simulink model "ee_motor_pmsm_drive_noContr"  (R2021b)
settings: Solver=ode23t  StartTime=0.0  StopTime=tsim  FixedStep=Ts  MaxStep=1e-6  RelTol=1e-4  AbsTol=1e-3  EnableMultiTasking=on
values from neighbouring files (symbols this model uses):
  angleVec = [0 1 2 3 4 5 6 7 8 9 10 11 ... (31 elements, 1x31)]    [currentsDQ_LUT.mat]    (also in di_pmsm_model_generator.m = [0:1:90]; di_pmsm_model_motor.m = [0:1:90])
  fsw = 2e3    (= 2000)    [ee_motor_pmsm_drive_noContr_params.m]    (also in ee_motor_pmsm_drive_test_params.m = 20000)
  Imax = 1000    [ee_motor_pmsm_drive_noContr_params.m]    (also in ee_motor_pmsm_drive_test_params.m = 320)
  J = 0.02    [di_pmsm_model_MPC.m]    (also in di_pmsm_model_generator_invLUT_V2.m; ee_motor_pmsm_drive_noContr_params.m)
  Ld = 0.0013    [di_pmsm_model_MPC.m]    (also in di_pmsm_model_generator_idealMod.m = (mean(dflux(p60_idx,:))-mean(dflux(m90_idx,:)))/(60-(-90)); ee_4d_table.m = 0.0002; ee_motor_pmsm_drive_noContr_params.m; ee_motor_pmsm_drive_test_params.m)
  Lq = 0.0039    [di_pmsm_model_MPC.m]    (also in di_pmsm_model_generator_idealMod.m = (mean(fq(p30_idx,:))-mean(fq(m30_idx,:)))/(30-(-30)); ee_4d_table.m = 0.0005; ee_motor_pmsm_drive_noContr_params.m; ee_motor_pmsm_drive_test_params.m)
  N = 4    [ee_4d_table.m]    (also in flux_derivatives_test.m = 6)
  PM = 0.1571    [di_pmsm_model_MPC.m]    (also in di_pmsm_model_generator_idealMod.m = fd_0; ee_4d_table.m = 0.1; ee_motor_pmsm_drive_noContr_params.m; ee_motor_pmsm_drive_test_params.m)
  rpm0 = 7200    [ee_motor_pmsm_drive_noContr_params.m]    (also in ee_motor_pmsm_drive_test_params.m = rpm_nom)
  Rs = 0.013    [ee_4d_table.m]    (also in ee_motor_pmsm_drive_noContr_params.m = 0.07; ee_motor_pmsm_drive_test_params.m = 0.07; flux_derivatives_test.m)
  Tmax = 460    [di_pmsm_model_MPC.m]    (also in ee_motor_pmsm_drive_noContr_params.m = 1.5*N*PM*Imax; ee_motor_pmsm_drive_test_params.m = 1.5*N*PM*Imax)
  torque = [461.04655919 409.33694322 395.67421775 372.972407 342.22869649 310.06846718 277.66285866 246.48195035 220.59637081 202.25585677 184.09571331 161.22594217 ... (40131 elements, 21x21x91)]    [torqueDQ_LUT_new.mat]
  torque0 = 0    [ee_motor_pmsm_drive_noContr_params.m]    (also in ee_motor_pmsm_drive_test_params.m)
  Ts = 1e-6    (= 1e-06)    [PruebaRN.m]    (also in di_pmsm_model_generator.m; di_pmsm_model_generator_idealMod.m; di_pmsm_model_generator_invLUT.m; di_pmsm_model_generator_invLUT_V2.m)
  Tsc = 1/fc    (= 5e-05)    [ee_motor_pmsm_drive_noContr_params.m]    (also in ee_motor_pmsm_drive_test_params.m = 5e-06)
  Vdc = 50    [ee_motor_pmsm_drive_noContr_params.m]
undefined symbols (not defined in the file or in its folder): data, idVec, iqVec, kif, kin, kit, kpf, kpn, kpt, vpor
libraries: simulink_need_slupdate x3, eeTransforms x3, slpidlib x3, eePwmGeneratorTwoLevel x1, simulink x1
Description:
  | HEV PMSM Drive Test Harness
settings Model: Creator=The MathWorks, Inc.  LastModifiedBy=crist
settings SolverCC: AutoScaleAbsTol=off  MaxConsecutiveMinStep=2  AlgebraicLoopSolver=TrustRegion
settings DataIOCC: LimitDataPoints=on  MaxDataPoints=35000  SaveFormat=StructureWithTime  SaveOutput=off  DSMLogging=off  ReturnWorkspaceOutputs=off  SignalLoggingName=logsout_ee_motor_pmsm_drive
settings OptimizationCC: LifeSpan=inf
settings DebuggingCC: UnderspecifiedInitializationDetection=Classic  MergeDetectMultiDrivingBlocksExec=none  AllowSymbolicDim=off  PregeneratedLibrarySubsystemCodeDiagnostic=none  SFUnexpectedBacktrackingDiag=warning  SFNoUnconditionalDefaultTransitionDiag=warning  SFExecutionAtInitializationDiag=none  SFMachineParentedDataDiag=warning  ArithmeticOperatorsInVariantConditions=warning
settings HardwareCC: ProdBitPerPointer=32  ProdBitPerSizeT=32  ProdBitPerPtrDiffT=32  ProdLargestAtomicFloat=None  ProdIntDivRoundTo=Undefined  ProdEndianess=Unspecified  ProdWordSize=32  ProdHWDeviceType=32-bit Generic
settings ModelReferenceCC: PropagateSignalLabelsOutOfModel=off
settings SFSimCC: SimUseLocalCustomCode=off
settings RTWCC: RTWUseLocalCustomCode=off
settings CodeAppCC: StateflowObjectComments=on
settings GRTTargetCC: TargetLangStandard=C89/C90 (ANSI)
settings ConfigComp: CovMetricSettings=dw  CovSaveCumulativeToWorkspaceVar=on  CovSaveSingleToWorkspaceVar=on  CovExternalEMLEnable=off  CovSFcnEnable=off
settings SimscapeCC: SimscapeLogType=all  SimscapeLogSimulationStatistics=on  SimscapeLogName=simlog_ee_motor_pmsm_drive  SimscapeLogDecimation=10  SimscapeLogLimitData=off  SimscapeLogDataHistory=1000000

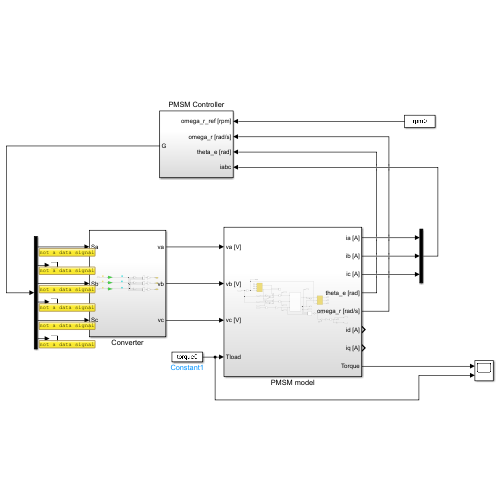
[thumbnail: Simulink's stored preview of the top-level diagram]
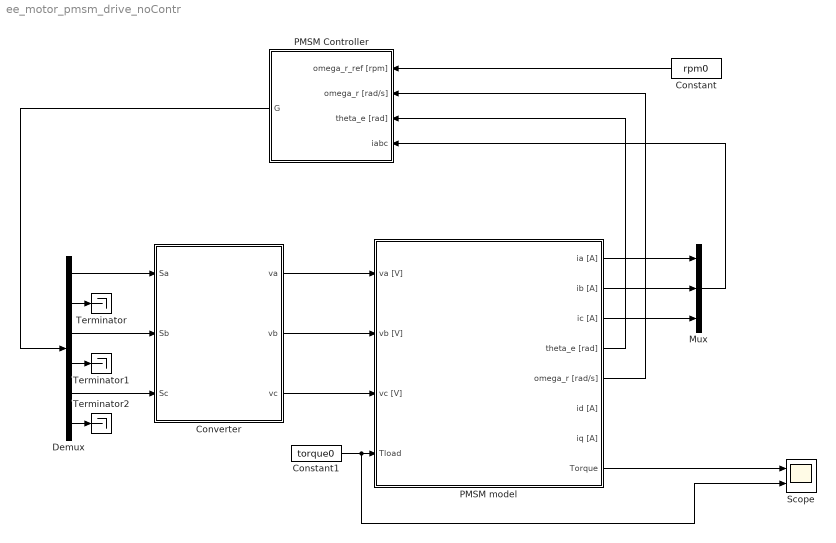
== system ee_motor_pmsm_drive_noContr ==
  Constant : Constant  Value=rpm0
  Constant1 : Constant  Value=torque0
  Converter : Subsystem
  Demux : Demux  Outputs=6
  Mux : Mux  Inputs=3
  PMSM Controller : Subsystem
  PMSM model : Subsystem
  Scope : Scope  NumInputPorts=2
  Terminator : Terminator
  Terminator1 : Terminator
  Terminator2 : Terminator
  wires:
  PMSM model/2(ib [A]) -> Mux/2
  PMSM model/1(ia [A]) -> Mux/1
  PMSM model/3(ic [A]) -> Mux/3
  Mux/1 -> PMSM Controller/4(iabc)
  Constant1/1 -> Scope/2, PMSM model/4(Tload)
  Constant/1 -> PMSM Controller/1(omega_r_ref [rpm])
  PMSM model/5(omega_r [rad/s]) -> PMSM Controller/2(omega_r [rad/s])
  PMSM model/4(theta_e [rad]) -> PMSM Controller/3(theta_e [rad])
  Converter/1(va) -> PMSM model/1(va [V])
  Converter/3(vc) -> PMSM model/3(vc [V])
  Converter/2(vb) -> PMSM model/2(vb [V])
  Demux/1 -> Converter/1(Sa)
  PMSM Controller/1(G) -> Demux/1
  Demux/3 -> Converter/2(Sb)
  Demux/5 -> Converter/3(Sc)
  Demux/2 -> Terminator/1
  Demux/4 -> Terminator1/1
  Demux/6 -> Terminator2/1
  PMSM model/8(Torque) -> Scope/1

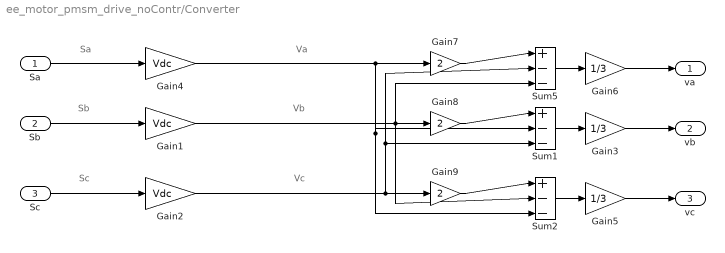
== system ee_motor_pmsm_drive_noContr/Converter ==
  note: Vb
  note: Sa
  note: Sc
  note: Va
  note: Vc
  note: Sb
  Sa : Inport
  Sb : Inport  Port=2
  Sc : Inport  Port=3
  Gain1 : Gain  Gain=Vdc
  Gain2 : Gain  Gain=Vdc
  Gain3 : Gain  Gain=1/3
  Gain4 : Gain  Gain=Vdc
  Gain5 : Gain  Gain=1/3
  Gain6 : Gain  Gain=1/3
  Gain7 : Gain  Gain=2
  Gain8 : Gain  Gain=2
  Gain9 : Gain  Gain=2
  Sum1 : Sum  Inputs=|+--
  Sum2 : Sum  Inputs=|+--
  Sum5 : Sum  Inputs=|+--
  va : Outport
  vb : Outport  Port=2
  vc : Outport  Port=3
  wires:
  Gain2/1 -> Gain9/1, Sum5/2, Sum1/3
  Gain9/1 -> Sum2/1
  Sum2/1 -> Gain5/1
  Gain4/1 -> Gain7/1, Sum1/2, Sum2/3
  Sum5/1 -> Gain6/1
  Gain7/1 -> Sum5/1
  Gain8/1 -> Sum1/1
  Sb/1 -> Gain1/1
  Gain6/1 -> va/1
  Gain5/1 -> vc/1
  Sum1/1 -> Gain3/1
  Gain3/1 -> vb/1
  Sc/1 -> Gain2/1
  Sa/1 -> Gain4/1
  Gain1/1 -> Gain8/1, Sum5/3, Sum2/2

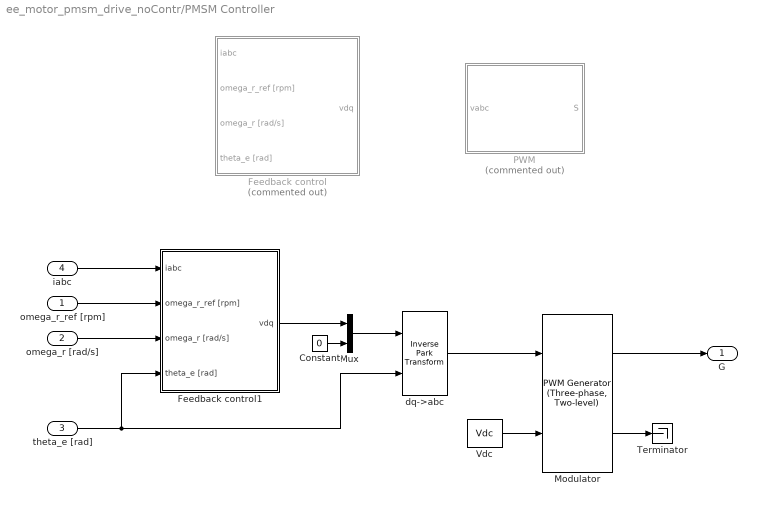
== system ee_motor_pmsm_drive_noContr/PMSM Controller ==
  omega_r_ref [rpm] : Inport
  omega_r [rad/s] : Inport  Port=2
  theta_e [rad] : Inport  Port=3
  iabc : Inport  Port=4
  Constant : Constant  Value=0  SampleTime=-1
  Feedback control : Subsystem  Commented=on
  Feedback control1 : Subsystem
  Modulator : eePwmGeneratorTwoLevel/PWM Generator (Three-phase, Two-level)  PWMMode=Continuous PWM (CPWM)  CPWMMode=SPWM: sinusoidal PWM  DPWMMode=60 DPWM: 60 degree discontinuous PWM  fsw=fsw  Ts=Ts
      settings: SourceProductBaseCode=PS
  Mux : Mux  Inputs=2
  PWM : Subsystem  Commented=on
  Terminator : Terminator
  Vdc : Constant  Value=Vdc  SampleTime=Tsc
  dq->abc : eeTransforms/Inverse Park Transform  AxisAlignment=Q-axis  PowerInvariant=off
  G : Outport  VectorParamsAs1DForOutWhenUnconnected=off
  wires:
  Vdc/1 -> Modulator/2
  Modulator/2 -> Terminator/1
  Modulator/1 -> G/1
  Constant/1 -> Mux/2
  Mux/1 -> dq->abc/1
  dq->abc/1 -> Modulator/1
  theta_e [rad]/1 -> Feedback control1/4(theta_e [rad]), dq->abc/2
  Feedback control1/1(vdq) -> Mux/1
  iabc/1 -> Feedback control1/1(iabc)
  omega_r_ref [rpm]/1 -> Feedback control1/2(omega_r_ref [rpm])
  omega_r [rad/s]/1 -> Feedback control1/3(omega_r [rad/s])

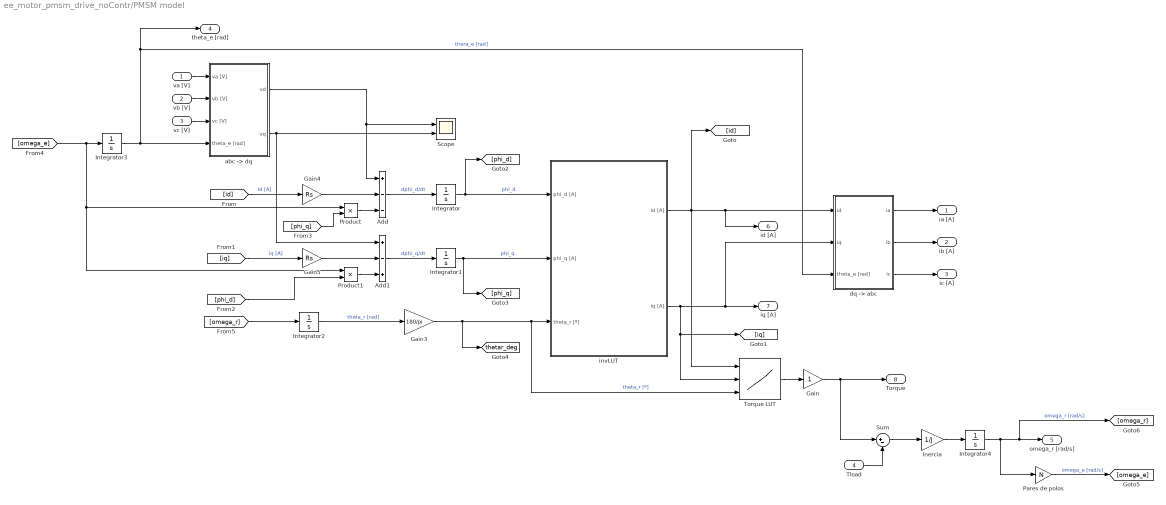
== system ee_motor_pmsm_drive_noContr/PMSM model ==
  va [V] : Inport
  vb [V] : Inport  Port=2
  vc [V] : Inport  Port=3
  Tload : Inport  Port=4
  Add : Sum  Inputs=+--
  Add1 : Sum  Inputs=+-+
  Gain : Gain
  Gain3 : Gain  Gain=180/pi
  Gain4 : Gain  Gain=Rs
  Gain5 : Gain  Gain=Rs
  Inercia : Gain  Gain=1/J
  Integrator : Integrator  InitialCondition=-0.2
  Integrator1 : Integrator
  Integrator2 : Integrator  WrapState=on  WrappedStateUpperValue=2*pi/3/N  WrappedStateLowerValue=0
  Integrator3 : Integrator
  Integrator4 : Integrator  InitialCondition=750
  Pares de polos : Gain  Gain=N
  Product : Product
  Product1 : Product
  Scope : Scope  NumInputPorts=2
  Sum : Sum  Inputs=|+-
  Torque LUT : Lookup_n-D  NumberOfTableDimensions=3  LookupTableObject=iD  BreakpointsForDimension1=idVec  BreakpointsForDimension2=iqVec  BreakpointsForDimension3=angleVec  Table=torque  InternalRulePriority=Speed  RndMeth=Simplest  InputSameDT=on
      settings: InputPortMap=u0,u1,u2
  "abc -> dq" : Subsystem
  "dq -> abc" : Subsystem
  "invLUT " : Subsystem
  ia [A] : Outport
  ib [A] : Outport  Port=2
  ic [A] : Outport  Port=3
  theta_e [rad] : Outport  Port=4
  omega_r [rad/s] : Outport  Port=5
  id [A] : Outport  Port=6
  iq [A] : Outport  Port=7
  Torque : Outport  Port=8
  tag scope: thetar_deg=global
  wires:
  Product/1 -> Add/3
  Integrator1/1 -> [phi_q], "invLUT "/2(phi_q [A])  "phi_q"
  [phi_q] -> Product/2
  [omega_e] -> Product/1, Product1/1, Integrator3/1
  Add/1 -> Integrator/1  "dphi_d/dt"
  [id] -> Gain4/1  "id [A]"
  Product1/1 -> Add1/3
  "invLUT "/1(id [A]) -> "dq -> abc"/1(id), id [A]/1, Torque LUT/1, [id]
  Integrator/1 -> "invLUT "/1(phi_d [A]), [phi_d]  "phi_d"
  "invLUT "/2(iq [A]) -> Torque LUT/2, [iq], "dq -> abc"/2(iq), iq [A]/1
  Add1/1 -> Integrator1/1  "dphi_q/dt"
  Gain5/1 -> Add1/2
  Gain4/1 -> Add/2
  "abc -> dq"/2(vq) -> Add1/1, Scope/2
  [iq] -> Gain5/1  "iq [A]"
  [phi_d] -> Product1/2
  "abc -> dq"/1(vd) -> Scope/1, Add/1
  va [V]/1 -> "abc -> dq"/1(va [V])
  vb [V]/1 -> "abc -> dq"/2(vb [V])
  vc [V]/1 -> "abc -> dq"/3(vc [V])
  Gain3/1 -> [thetar_deg], Torque LUT/3, "invLUT "/3(theta_r [º])  "theta_r [º]"
  [omega_r] -> Integrator2/1
  "dq -> abc"/1(ia) -> ia [A]/1
  "dq -> abc"/2(ib) -> ib [A]/1
  "dq -> abc"/3(ic) -> ic [A]/1
  Integrator2/1 -> Gain3/1  "theta_r [rad]"
  Integrator3/1 -> theta_e [rad]/1, "dq -> abc"/3(theta_e [rad]), "abc -> dq"/4(theta_e [rad])  "thera_e [rad]"
  Gain/1 -> Torque/1, Sum/1
  Pares de polos/1 -> [omega_e]  "omega_e [rad/s]"
  Sum/1 -> Inercia/1
  Inercia/1 -> Integrator4/1
  Integrator4/1 -> omega_r [rad/s]/1, [omega_r], Pares de polos/1  "omega_r [rad/s]"
  Tload/1 -> Sum/2
  Torque LUT/1 -> Gain/1

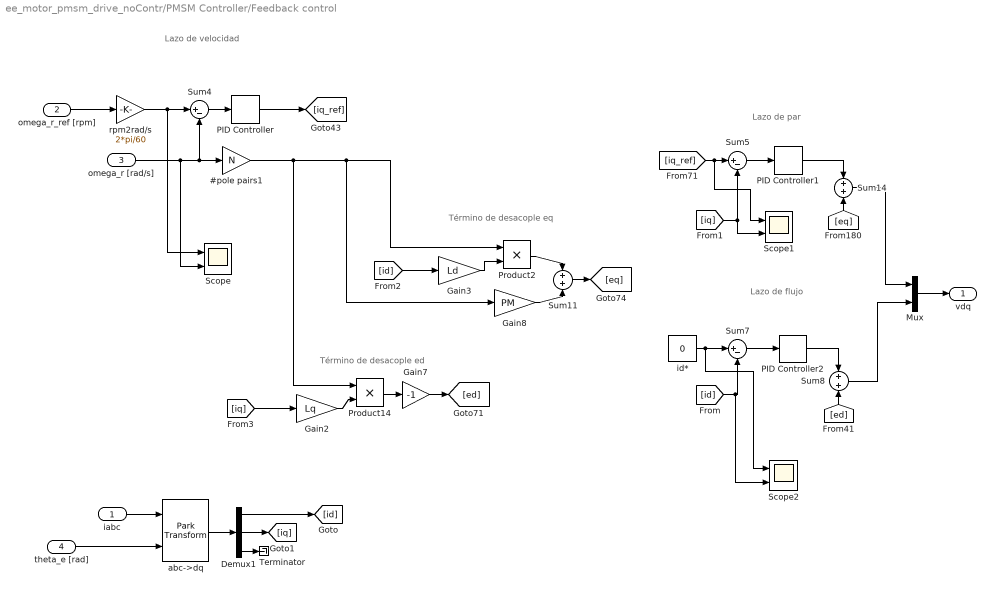
== system ee_motor_pmsm_drive_noContr/PMSM Controller/Feedback control ==
  note: Término de desacople eq
  note: Lazo de flujo
  note: Término de desacople ed
  note: Lazo de par
  note: Lazo de velocidad
  iabc : Inport
  omega_r_ref [rpm] : Inport  Port=2
  omega_r [rad/s] : Inport  Port=3
  theta_e [rad] : Inport  Port=4
  #pole pairs1 : Gain  Gain=N
  Demux1 : Demux  Outputs=3
  Gain2 : Gain  Gain=Lq
  Gain3 : Gain  Gain=Ld
  Gain7 : Gain  Gain=-1
  Gain8 : Gain  Gain=PM
  Mux : Mux  Inputs=2
  PID Controller : simulink_need_slupdate/PID Controller  P=kpn  I=kin  D=0
  PID Controller1 : simulink_need_slupdate/PID Controller  P=kpt  I=kit  D=0
  PID Controller2 : simulink_need_slupdate/PID Controller  P=kpf  I=kif  D=0
  Product14 : Product  RndMeth=Zero
  Product2 : Product  RndMeth=Zero
  Scope : Scope  NumInputPorts=2
  Scope1 : Scope  NumInputPorts=2
  Scope2 : Scope  NumInputPorts=2
  Sum11 : Sum
  Sum14 : Sum
  Sum4 : Sum  Inputs=|+-
  Sum5 : Sum  Inputs=|+-
  Sum7 : Sum  Inputs=|+-
  Sum8 : Sum
  Terminator : Terminator
  abc->dq : eeTransforms/Park Transform  AxisAlignment=Q-axis  PowerInvariant=off
  id* : Constant  Value=0  SampleTime=Tsc
  rpm2rad/s : Gain  Gain=2*pi/60
  vdq : Outport
  wires:
  abc->dq/1 -> Demux1/1
  iabc/1 -> abc->dq/1
  omega_r_ref [rpm]/1 -> rpm2rad/s/1
  Demux1/3 -> Terminator/1
  theta_e [rad]/1 -> abc->dq/2
  Sum4/1 -> PID Controller/1
  PID Controller1/1 -> Sum14/1
  Product14/1 -> Gain7/1
  Sum5/1 -> PID Controller1/1
  [eq] -> Sum14/2
  #pole pairs1/1 -> Product14/1, Gain8/1, Product2/1
  Sum11/1 -> [eq]
  id*/1 -> Scope2/1, Sum7/1
  Gain8/1 -> Sum11/2
  [ed] -> Sum8/2
  PID Controller/1 -> [iq_ref]
  Gain7/1 -> [ed]
  Gain2/1 -> Product14/2
  Sum7/1 -> PID Controller2/1
  PID Controller2/1 -> Sum8/1
  [iq_ref] -> Scope1/1, Sum5/1
  Gain3/1 -> Product2/2
  Product2/1 -> Sum11/1
  Sum8/1 -> Mux/2
  Sum14/1 -> Mux/1
  rpm2rad/s/1 -> Scope/1, Sum4/1
  omega_r [rad/s]/1 -> Scope/2, #pole pairs1/1, Sum4/2
  [id] -> Scope2/2, Sum7/2
  [iq] -> Sum5/2, Scope1/2
  [id] -> Gain3/1
  Demux1/1 -> [id]
  [iq] -> Gain2/1
  Demux1/2 -> [iq]
  Mux/1 -> vdq/1

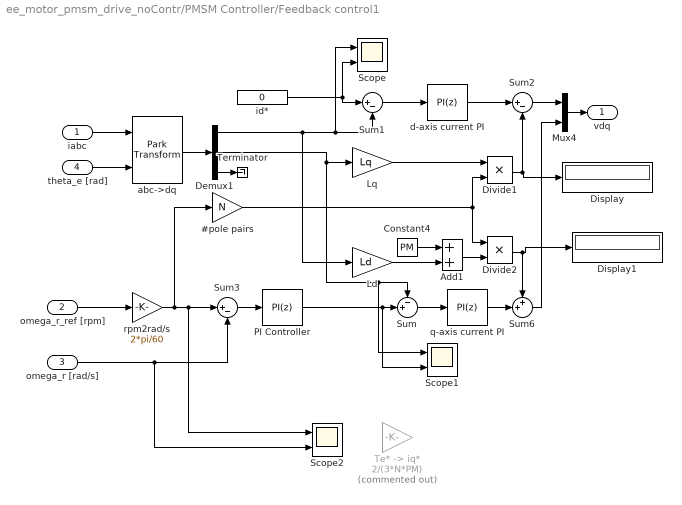
== system ee_motor_pmsm_drive_noContr/PMSM Controller/Feedback control1 ==
  iabc : Inport
  omega_r_ref [rpm] : Inport  Port=2
  omega_r [rad/s] : Inport  Port=3
  theta_e [rad] : Inport  Port=4
  #pole pairs : Gain  Gain=N
  Add1 : Sum
  Constant4 : Constant  Value=PM  SampleTime=-1
  Demux1 : Demux  Outputs=3
  Display : Display
  Display1 : Display
  Divide1 : Product  Inputs=**
  Divide2 : Product  Inputs=**
  Ld : Gain  Gain=Ld
  Lq : Gain  Gain=Lq
  Mux4 : Mux  Inputs=2
  PI Controller : slpidlib/PID Controller  Controller=PI  Form=Parallel  TimeDomain=Discrete-time  UseExternalTs=off  SampleTime=Tsc  IntegratorMethod=Forward Euler  FilterMethod=Forward Euler  ControllerParametersSource=internal  P=1  I=1  D=0  UseFilter=on  N=100  TunerSelectOption=Transfer Function Based (PID Tuner App)  InitialConditionSource=internal  InitialConditionForIntegrator=0  InitialConditionForFilter=0  DifferentiatorICPrevScaledInput=0  ExternalReset=none  TrackingMode=off  Kt=1  LimitOutput=off  SatLimitsSource=internal  UpperSaturationLimit=Tmax*1.5  LowerSaturationLimit=-Tmax*1.5  LinearizeAsGain=on  AntiWindupMode=back-calculation  Kb=1000  POutMin=[]  POutMax=[]  IOutMin=[]  IOutMax=[]  DOutMin=[]  DOutMax=[]  NOutMin=[]  NOutMax=[]  SumOutMin=[]  SumOutMax=[]  SaturationOutMin=[]  SaturationOutMax=[]  PParamMin=[]  PParamMax=[]  IParamMin=[]  IParamMax=[]  DParamMin=[]  DParamMax=[]  NParamMin=[]  NParamMax=[]  KbParamMin=[]  KbParamMax=[]  KtParamMin=[]  KtParamMax=[]  KbOutMin=[]  KbOutMax=[]  KtOutMin=[]  KtOutMax=[]  IntegratorOutMin=[]  IntegratorOutMax=[]  FilterOutMin=[]  FilterOutMax=[]  SumI1OutMin=[]  SumI1OutMax=[]  SumI2OutMin=[]  SumI2OutMax=[]  SumI3OutMin=[]  SumI3OutMax=[]  SumI4OutMin=[]  SumI4OutMax=[]  SumDOutMin=[]  SumDOutMax=[]  DifferentiatorOutMin=[]  DifferentiatorOutMax=[]  FilterDiffOutCoefMin=[]  FilterDiffOutCoefMax=[]  ReciprocalOutMin=[]  ReciprocalOutMax=[]  SumDenOutMin=[]  SumDenOutMax=[]  SumNumOutMin=[]  SumNumOutMax=[]  DivideOutMin=[]  DivideOutMax=[]  UdiffTsProdOutMin=[]  UdiffTsProdOutMax=[]  NTsProdOutMin=[]  NTsProdOutMax=[]  UintegralTsProdOutMin=[]  UintegralTsProdOutMax=[]  UngainTsProdOutMin=[]  UngainTsProdOutMax=[]  IntegratorContinuousStateAttributes=''  IntegratorStateMustResolveToSignalObject=off  IntegratorRTWStateStorageClass=Auto  FilterContinuousStateAttributes=''  FilterStateMustResolveToSignalObject=off  FilterRTWStateStorageClass=Auto  ParallelPVariant=InternalParameters  IdealPVariant=Disabled  IVariant=InternalParameters  DVariant=Disabled  IntegratorVariant=Discrete  SatVariant=Disabled  AWVariant=Passthrough  PCopyVariant=Disabled  TRVariant=Disabled  FdbkBlocksVariant=Forward  IdealPFdbkVariant=Disabled  SatFdbkVariant=Disabled  DerivativeFilterVariant=Disabled  NVariant=Disabled  NCopyVariant=Disabled_SignalSpec  FilterICVariant=Disabled  IntegratorICVariant=InternalICs  ExternalResetVariant=Disabled  TRSumVariant=Passthrough  SumFdbkVariant=Disabled  SumVariant=Sum_PI  TsampFilterVariant=InternalTs  TsampNgainVariant=Passthrough  TsampIntegralVariant=Passthrough  ExternalSaturationOutDataTypeStr=Inherit: Same as second input
  Scope : Scope  NumInputPorts=2
  Scope1 : Scope  NumInputPorts=2
  Scope2 : Scope  NumInputPorts=2
  Sum : Sum  Inputs=-+|
  Sum1 : Sum  Inputs=|+-
  Sum2 : Sum  Inputs=|+-
  Sum3 : Sum  Inputs=|+-
  Sum6 : Sum  Inputs=++|
  "Te* -> iq*" : Gain  Commented=on  Gain=2/(3*N*PM)
  Terminator : Terminator
  abc->dq : eeTransforms/Park Transform  AxisAlignment=Q-axis  PowerInvariant=off
  d-axis current PI : slpidlib/PID Controller  Controller=PI  Form=Parallel  TimeDomain=Discrete-time  UseExternalTs=off  SampleTime=Tsc  IntegratorMethod=Forward Euler  FilterMethod=Forward Euler  ControllerParametersSource=internal  P=1  I=10  D=0  UseFilter=on  N=100  TunerSelectOption=Transfer Function Based (PID Tuner App)  InitialConditionSource=internal  InitialConditionForIntegrator=0  InitialConditionForFilter=0  DifferentiatorICPrevScaledInput=0  ExternalReset=none  TrackingMode=off  Kt=1  LimitOutput=on  SatLimitsSource=internal  UpperSaturationLimit=5*Rs*Imax  LowerSaturationLimit=-5*Rs*Imax  LinearizeAsGain=on  AntiWindupMode=back-calculation  Kb=1000  POutMin=[]  POutMax=[]  IOutMin=[]  IOutMax=[]  DOutMin=[]  DOutMax=[]  NOutMin=[]  NOutMax=[]  SumOutMin=[]  SumOutMax=[]  SaturationOutMin=[]  SaturationOutMax=[]  PParamMin=[]  PParamMax=[]  IParamMin=[]  IParamMax=[]  DParamMin=[]  DParamMax=[]  NParamMin=[]  NParamMax=[]  KbParamMin=[]  KbParamMax=[]  KtParamMin=[]  KtParamMax=[]  KbOutMin=[]  KbOutMax=[]  KtOutMin=[]  KtOutMax=[]  IntegratorOutMin=[]  IntegratorOutMax=[]  FilterOutMin=[]  FilterOutMax=[]  SumI1OutMin=[]  SumI1OutMax=[]  SumI2OutMin=[]  SumI2OutMax=[]  SumI3OutMin=[]  SumI3OutMax=[]  SumI4OutMin=[]  SumI4OutMax=[]  SumDOutMin=[]  SumDOutMax=[]  DifferentiatorOutMin=[]  DifferentiatorOutMax=[]  FilterDiffOutCoefMin=[]  FilterDiffOutCoefMax=[]  ReciprocalOutMin=[]  ReciprocalOutMax=[]  SumDenOutMin=[]  SumDenOutMax=[]  SumNumOutMin=[]  SumNumOutMax=[]  DivideOutMin=[]  DivideOutMax=[]  UdiffTsProdOutMin=[]  UdiffTsProdOutMax=[]  NTsProdOutMin=[]  NTsProdOutMax=[]  UintegralTsProdOutMin=[]  UintegralTsProdOutMax=[]  UngainTsProdOutMin=[]  UngainTsProdOutMax=[]  IntegratorContinuousStateAttributes=''  IntegratorStateMustResolveToSignalObject=off  IntegratorRTWStateStorageClass=Auto  FilterContinuousStateAttributes=''  FilterStateMustResolveToSignalObject=off  FilterRTWStateStorageClass=Auto  ParallelPVariant=InternalParameters  IdealPVariant=Disabled  IVariant=InternalParameters  DVariant=Disabled  IntegratorVariant=Discrete  SatVariant=Enabled  AWVariant=BackCalculation  PCopyVariant=Disabled  TRVariant=Disabled  FdbkBlocksVariant=Forward  IdealPFdbkVariant=Disabled  SatFdbkVariant=Disabled  DerivativeFilterVariant=Disabled  NVariant=Disabled  NCopyVariant=Disabled_SignalSpec  FilterICVariant=Disabled  IntegratorICVariant=InternalICs  ExternalResetVariant=Disabled  TRSumVariant=Passthrough  SumFdbkVariant=Disabled  SumVariant=Sum_PI  TsampFilterVariant=InternalTs  TsampNgainVariant=Passthrough  TsampIntegralVariant=Passthrough  ExternalSaturationOutDataTypeStr=Inherit: Same as second input
  id* : Constant  Value=0  SampleTime=Tsc
  q-axis current PI : slpidlib/PID Controller  Controller=PI  Form=Parallel  TimeDomain=Discrete-time  UseExternalTs=off  SampleTime=Tsc  IntegratorMethod=Forward Euler  FilterMethod=Forward Euler  ControllerParametersSource=internal  P=50  I=100  D=0.000539029417831173  UseFilter=on  N=29631.0341187165  TunerSelectOption=Transfer Function Based (PID Tuner App)  InitialConditionSource=internal  InitialConditionForIntegrator=0  InitialConditionForFilter=0  DifferentiatorICPrevScaledInput=0  ExternalReset=none  TrackingMode=off  Kt=1  LimitOutput=on  SatLimitsSource=internal  UpperSaturationLimit=5*Rs*Imax  LowerSaturationLimit=-5*Rs*Imax  LinearizeAsGain=on  AntiWindupMode=back-calculation  Kb=1000  POutMin=[]  POutMax=[]  IOutMin=[]  IOutMax=[]  DOutMin=[]  DOutMax=[]  NOutMin=[]  NOutMax=[]  SumOutMin=[]  SumOutMax=[]  SaturationOutMin=[]  SaturationOutMax=[]  PParamMin=[]  PParamMax=[]  IParamMin=[]  IParamMax=[]  DParamMin=[]  DParamMax=[]  NParamMin=[]  NParamMax=[]  KbParamMin=[]  KbParamMax=[]  KtParamMin=[]  KtParamMax=[]  KbOutMin=[]  KbOutMax=[]  KtOutMin=[]  KtOutMax=[]  IntegratorOutMin=[]  IntegratorOutMax=[]  FilterOutMin=[]  FilterOutMax=[]  SumI1OutMin=[]  SumI1OutMax=[]  SumI2OutMin=[]  SumI2OutMax=[]  SumI3OutMin=[]  SumI3OutMax=[]  SumI4OutMin=[]  SumI4OutMax=[]  SumDOutMin=[]  SumDOutMax=[]  DifferentiatorOutMin=[]  DifferentiatorOutMax=[]  FilterDiffOutCoefMin=[]  FilterDiffOutCoefMax=[]  ReciprocalOutMin=[]  ReciprocalOutMax=[]  SumDenOutMin=[]  SumDenOutMax=[]  SumNumOutMin=[]  SumNumOutMax=[]  DivideOutMin=[]  DivideOutMax=[]  UdiffTsProdOutMin=[]  UdiffTsProdOutMax=[]  NTsProdOutMin=[]  NTsProdOutMax=[]  UintegralTsProdOutMin=[]  UintegralTsProdOutMax=[]  UngainTsProdOutMin=[]  UngainTsProdOutMax=[]  IntegratorContinuousStateAttributes=''  IntegratorStateMustResolveToSignalObject=off  IntegratorRTWStateStorageClass=Auto  FilterContinuousStateAttributes=''  FilterStateMustResolveToSignalObject=off  FilterRTWStateStorageClass=Auto  ParallelPVariant=InternalParameters  IdealPVariant=Disabled  IVariant=InternalParameters  DVariant=Disabled  IntegratorVariant=Discrete  SatVariant=Enabled  AWVariant=BackCalculation  PCopyVariant=Disabled  TRVariant=Disabled  FdbkBlocksVariant=Forward  IdealPFdbkVariant=Disabled  SatFdbkVariant=Disabled  DerivativeFilterVariant=Disabled  NVariant=Disabled  NCopyVariant=Disabled_SignalSpec  FilterICVariant=Disabled  IntegratorICVariant=InternalICs  ExternalResetVariant=Disabled  TRSumVariant=Passthrough  SumFdbkVariant=Disabled  SumVariant=Sum_PI  TsampFilterVariant=InternalTs  TsampNgainVariant=Passthrough  TsampIntegralVariant=Passthrough  ExternalSaturationOutDataTypeStr=Inherit: Same as second input
  rpm2rad/s : Gain  Gain=2*pi/60
  vdq : Outport  VectorParamsAs1DForOutWhenUnconnected=off
  wires:
  abc->dq/1 -> Demux1/1
  Sum2/1 -> Mux4/1
  iabc/1 -> abc->dq/1
  Constant4/1 -> Add1/1
  Add1/1 -> Divide2/2
  Demux1/1 -> Ld/1, Sum1/2, Scope/1
  omega_r_ref [rpm]/1 -> rpm2rad/s/1
  d-axis current PI/1 -> Sum2/1
  Sum3/1 -> PI Controller/1
  Sum1/1 -> d-axis current PI/1
  Sum6/1 -> Mux4/2
  Ld/1 -> Add1/2
  #pole pairs/1 -> Divide2/1, Divide1/2
  Sum/1 -> q-axis current PI/1
  PI Controller/1 -> Scope1/2, Sum/2
  Divide2/1 -> Display1/1, Sum6/1
  q-axis current PI/1 -> Sum6/2
  Demux1/2 -> Scope1/1, Sum/1, Lq/1
  rpm2rad/s/1 -> #pole pairs/1, Scope2/1, Sum3/1
  omega_r [rad/s]/1 -> Scope2/2, Sum3/2
  Mux4/1 -> vdq/1
  Lq/1 -> Divide1/1
  Divide1/1 -> Display/1, Sum2/2
  Demux1/3 -> Terminator/1
  id*/1 -> Sum1/1, Scope/2
  theta_e [rad]/1 -> abc->dq/2

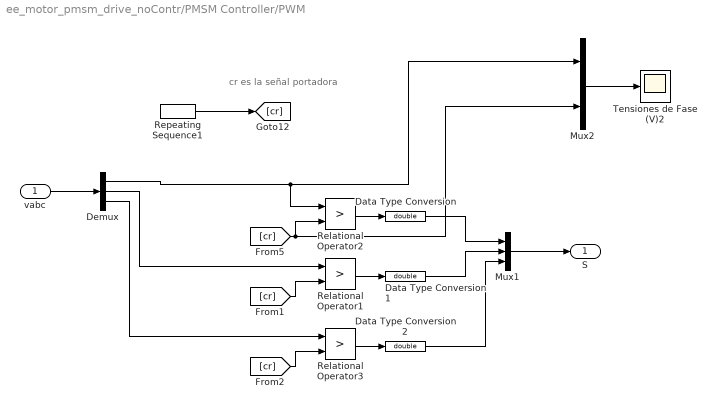
== system ee_motor_pmsm_drive_noContr/PMSM Controller/PWM ==
  note: cr es la señal portadora
  vabc : Inport
  Data Type Conversion : DataTypeConversion  OutDataTypeStr=double
  Data Type Conversion1 : DataTypeConversion  OutDataTypeStr=double
  Data Type Conversion2 : DataTypeConversion  OutDataTypeStr=double
  Demux : Demux  Outputs=3
  Mux1 : Mux  Inputs=3
  Mux2 : Mux  Inputs=2
  Relational Operator1 : RelationalOperator  Operator=>  OutDataTypeStr=boolean  RndMeth=Nearest
  Relational Operator2 : RelationalOperator  Operator=>  OutDataTypeStr=boolean  RndMeth=Nearest
  Relational Operator3 : RelationalOperator  Operator=>  OutDataTypeStr=boolean  RndMeth=Nearest
  Repeating Sequence1 : simulink/Sources/Repeating Sequence  rep_seq_t=[0 0.5/fsw 1/fsw]  rep_seq_y=[-vpor vpor -vpor]
  Tensiones de Fase (V)2 : Scope
  S : Outport
  wires:
  Relational Operator1/1 -> Data Type Conversion1/1
  [cr] -> Relational Operator3/2
  Data Type Conversion2/1 -> Mux1/3
  Data Type Conversion/1 -> Mux1/1
  Repeating Sequence1/1 -> [cr]
  Demux/2 -> Relational Operator1/1
  Data Type Conversion1/1 -> Mux1/2
  Relational Operator2/1 -> Data Type Conversion/1
  Demux/1 -> Mux2/1, Relational Operator2/1
  Demux/3 -> Relational Operator3/1
  [cr] -> Mux2/2, Relational Operator2/2
  Mux2/1 -> Tensiones de Fase (V)2/1
  [cr] -> Relational Operator1/2
  Relational Operator3/1 -> Data Type Conversion2/1
  vabc/1 -> Demux/1
  Mux1/1 -> S/1

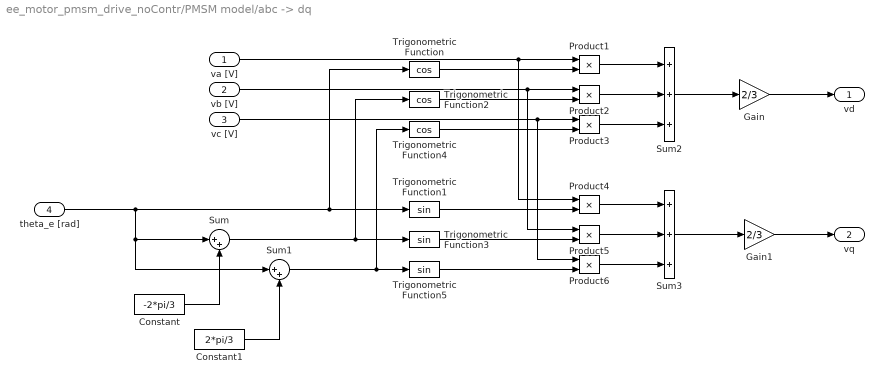
== system ee_motor_pmsm_drive_noContr/PMSM model/abc -> dq ==
  va [V] : Inport
  vb [V] : Inport  Port=2
  vc [V] : Inport  Port=3
  theta_e [rad] : Inport  Port=4
  Constant : Constant  Value=-2*pi/3
  Constant1 : Constant  Value=2*pi/3
  Gain : Gain  Gain=2/3
  Gain1 : Gain  Gain=2/3
  Product{1..6} (6 alike) : Product  RndMeth=Zero
  Sum : Sum  Inputs=|++
  Sum1 : Sum  Inputs=|++
  Sum2 : Sum  Inputs=+++
  Sum3 : Sum  Inputs=+++
  Trigonometric Function : Trigonometry  Operator=cos
  Trigonometric Function1 : Trigonometry
  Trigonometric Function2 : Trigonometry  Operator=cos
  Trigonometric Function3 : Trigonometry
  Trigonometric Function4 : Trigonometry  Operator=cos
  Trigonometric Function5 : Trigonometry
  vd : Outport
  vq : Outport  Port=2
  wires:
  Gain1/1 -> vq/1
  Gain/1 -> vd/1
  Product1/1 -> Sum2/1
  Trigonometric Function1/1 -> Product4/2
  vb [V]/1 -> Product5/1, Product2/1
  Trigonometric Function/1 -> Product1/2
  theta_e [rad]/1 -> Sum1/1, Sum/1, Trigonometric Function/1, Trigonometric Function1/1
  Sum2/1 -> Gain/1
  Sum3/1 -> Gain1/1
  Constant/1 -> Sum/2
  Constant1/1 -> Sum1/2
  Sum/1 -> Trigonometric Function3/1, Trigonometric Function2/1
  Sum1/1 -> Trigonometric Function4/1, Trigonometric Function5/1
  va [V]/1 -> Product4/1, Product1/1
  Product2/1 -> Sum2/2
  Product3/1 -> Sum2/3
  Product5/1 -> Sum3/2
  Product6/1 -> Sum3/3
  Product4/1 -> Sum3/1
  vc [V]/1 -> Product6/1, Product3/1
  Trigonometric Function2/1 -> Product2/2
  Trigonometric Function4/1 -> Product3/2
  Trigonometric Function3/1 -> Product5/2
  Trigonometric Function5/1 -> Product6/2

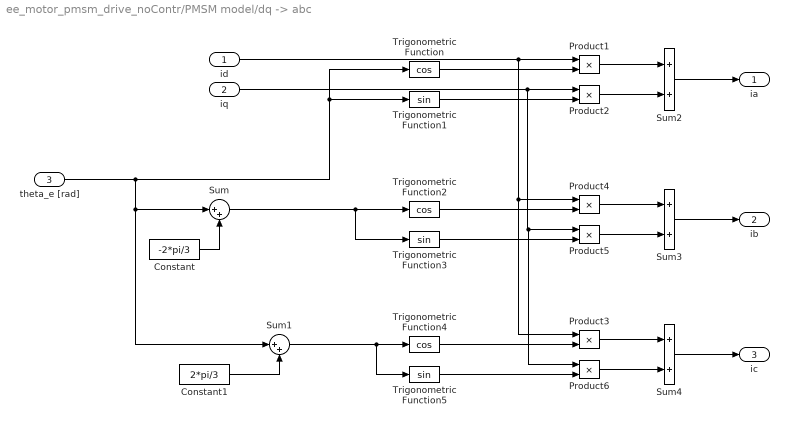
== system ee_motor_pmsm_drive_noContr/PMSM model/dq -> abc ==
  id : Inport
  iq : Inport  Port=2
  theta_e [rad] : Inport  Port=3
  Constant : Constant  Value=-2*pi/3
  Constant1 : Constant  Value=2*pi/3
  Product{1..6} (6 alike) : Product  RndMeth=Zero
  Sum : Sum  Inputs=|++
  Sum1 : Sum  Inputs=|++
  Sum2 : Sum
  Sum3 : Sum
  Sum4 : Sum
  Trigonometric Function : Trigonometry  Operator=cos
  Trigonometric Function1 : Trigonometry
  Trigonometric Function2 : Trigonometry  Operator=cos
  Trigonometric Function3 : Trigonometry
  Trigonometric Function4 : Trigonometry  Operator=cos
  Trigonometric Function5 : Trigonometry
  ia : Outport
  ib : Outport  Port=2
  ic : Outport  Port=3
  wires:
  Trigonometric Function3/1 -> Product5/2
  Trigonometric Function2/1 -> Product4/2
  Product4/1 -> Sum3/1
  Product5/1 -> Sum3/2
  Product2/1 -> Sum2/2
  id/1 -> Product1/1, Product3/1, Product4/1
  Sum1/1 -> Trigonometric Function5/1, Trigonometric Function4/1
  Sum/1 -> Trigonometric Function3/1, Trigonometric Function2/1
  Constant1/1 -> Sum1/2
  Constant/1 -> Sum/2
  theta_e [rad]/1 -> Sum/1, Sum1/1, Trigonometric Function1/1, Trigonometric Function/1
  Trigonometric Function/1 -> Product1/2
  iq/1 -> Product2/1, Product6/1, Product5/1
  Trigonometric Function1/1 -> Product2/2
  Product1/1 -> Sum2/1
  Sum2/1 -> ia/1
  Sum3/1 -> ib/1
  Sum4/1 -> ic/1
  Product6/1 -> Sum4/2
  Product3/1 -> Sum4/1
  Trigonometric Function4/1 -> Product3/2
  Trigonometric Function5/1 -> Product6/2

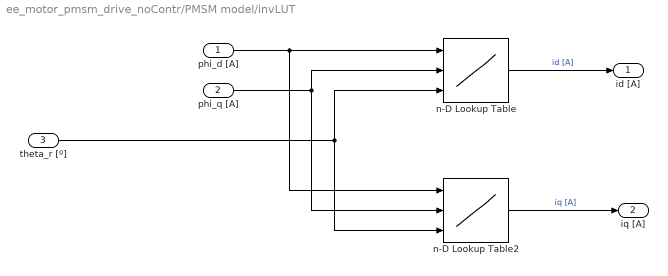
== system ee_motor_pmsm_drive_noContr/PMSM model/invLUT  ==
  phi_d [A] : Inport
  phi_q [A] : Inport  Port=2
  theta_r [º] : Inport  Port=3
  n-D Lookup Table : Lookup_n-D  NumberOfTableDimensions=3  LookupTableObject=iD  BreakpointsForDimension1=data.phi_d  BreakpointsForDimension2=data.phi_q  BreakpointsForDimension3=data.theta  Table=data.i_d  InternalRulePriority=Speed  RndMeth=Simplest  InputSameDT=on
      settings: InputPortMap=u0,u1,u2
  n-D Lookup Table2 : Lookup_n-D  NumberOfTableDimensions=3  LookupTableObject=iD  BreakpointsForDimension1=data.phi_d  BreakpointsForDimension2=data.phi_q  BreakpointsForDimension3=data.theta  Table=data.i_q  InternalRulePriority=Speed  RndMeth=Simplest  InputSameDT=on
      settings: InputPortMap=u0,u1,u2
  id [A] : Outport
  iq [A] : Outport  Port=2
  wires:
  n-D Lookup Table/1 -> id [A]/1  "id [A]"
  phi_d [A]/1 -> n-D Lookup Table2/1, n-D Lookup Table/1
  phi_q [A]/1 -> n-D Lookup Table2/2, n-D Lookup Table/2
  n-D Lookup Table2/1 -> iq [A]/1  "iq [A]"
  theta_r [º]/1 -> n-D Lookup Table2/3, n-D Lookup Table/3
